simulink model "sinc3_nplc_simulink"  (R2026a)
settings: Solver=FixedStepDiscrete  StopTime=0.5  FixedStep=5e-07
settings Model: Creator=jinwe  LastModifiedBy=jinwe

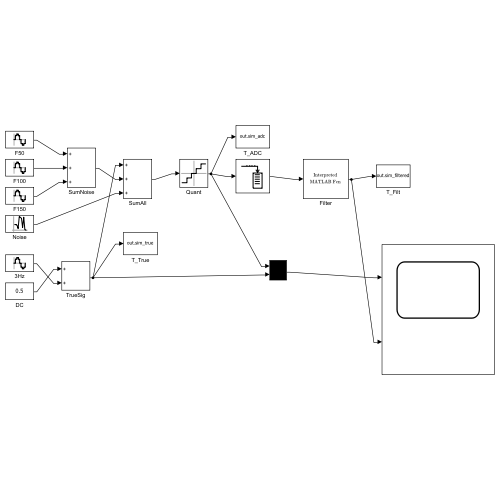
[thumbnail: Simulink's stored preview of the top-level diagram]
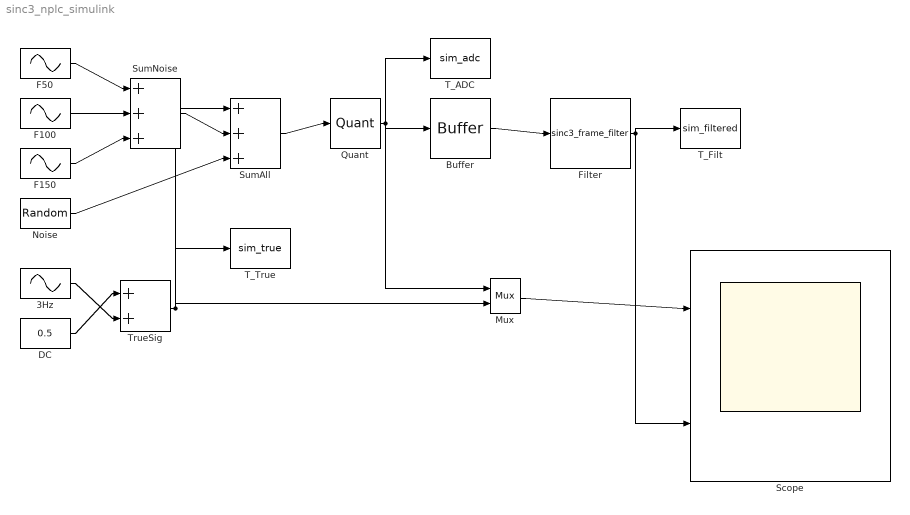
== system sinc3_nplc_simulink ==
  3Hz : Sin  Amplitude=0.05  Frequency=2*pi*3  SampleTime=5e-07
  Buffer : Buffer  N=40000
  DC : Constant  Value=0.5  SampleTime=5e-07
  F100 : Sin  Amplitude=0.3  Frequency=2*pi*100  SampleTime=5e-07
  F150 : Sin  Amplitude=0.1  Frequency=2*pi*150  SampleTime=5e-07
  F50 : Sin  Amplitude=1.0  Frequency=2*pi*50  SampleTime=5e-07
  Filter : MATLABFcn  MATLABFcn=sinc3_frame_filter  OutputDimensions=1
  Mux : Mux  Inputs=2
  Noise : RandomNumber  Variance=0.0004  SampleTime=5e-07
  Quant : Quantizer  QuantizationInterval=2/2^24
  Scope : Scope  NumInputPorts=2
  SumAll : Sum  Inputs=+++
  SumNoise : Sum  Inputs=+++
  T_ADC : ToWorkspace  VariableName=sim_adc  SampleTime=-1
  T_Filt : ToWorkspace  VariableName=sim_filtered  SampleTime=-1
  T_True : ToWorkspace  VariableName=sim_true  SampleTime=-1
  TrueSig : Sum
  wires:
  DC/1 -> TrueSig/1
  3Hz/1 -> TrueSig/2
  F50/1 -> SumNoise/1
  F100/1 -> SumNoise/2
  F150/1 -> SumNoise/3
  TrueSig/1 -> SumAll/1, T_True/1, Mux/2
  SumNoise/1 -> SumAll/2
  Noise/1 -> SumAll/3
  SumAll/1 -> Quant/1
  Quant/1 -> Buffer/1, T_ADC/1, Mux/1
  Buffer/1 -> Filter/1
  Filter/1 -> T_Filt/1, Scope/2
  Mux/1 -> Scope/1
